simulink model "PID_spring_2mass_damper_system"  (R2022b)
settings: Solver=FixedStepAuto  StartTime=0  StopTime=Tf  FixedStep=dt  RelTol=1e-3
values from neighbouring files (symbols this model uses):
  c1 = 1    [P_2mass__slx_main.m]
  c2 = 2    [P_2mass__slx_main.m]
  control_on = true    [P_2mass__slx_main.m]
  f1 = 60    [P_2mass__slx_main.m]
  f2 = 30    [P_2mass__slx_main.m]
  k1 = 10    [P_2mass__slx_main.m]
  k2 = 20    [P_2mass__slx_main.m]
  m1 = 1    [P_2mass__slx_main.m]
  m2 = 5    [P_2mass__slx_main.m]
  r = [0 0 0 0]'    [P_2mass__slx_main.m]
  v1 = 0    [P_2mass__slx_main.m]
  v2 = 0    [P_2mass__slx_main.m]
  x1 = 1    [P_2mass__slx_main.m]
  x2 = 2    [P_2mass__slx_main.m]
settings Model: Creator=murayama  LastModifiedBy=murayama
settings DataIOCC: SaveFormat=StructureWithTime  ReturnWorkspaceOutputs=off
settings OptimizationCC: BlockReduction=off  BufferReuse=off
settings DebuggingCC: AlgebraicLoopMsg=none

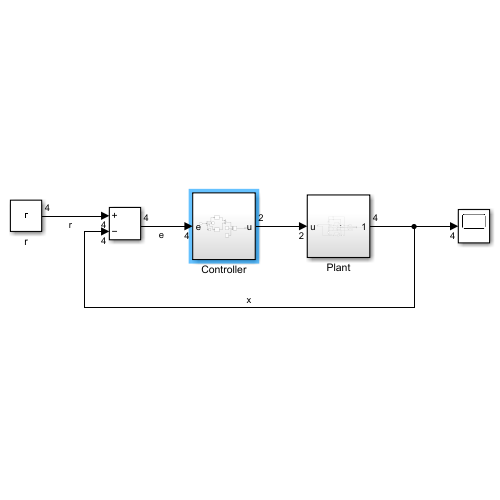
[thumbnail: Simulink's stored preview of the top-level diagram]
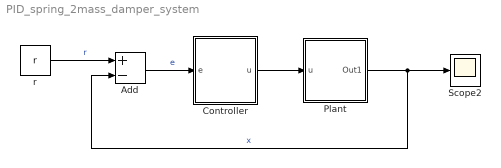
== system PID_spring_2mass_damper_system ==
  Add : Sum  Inputs=+-
  Controller : Subsystem
  Plant : Subsystem
  Scope2 : Scope
  r : Constant  Value=r
  wires:
  Plant/1(Out1) -> Scope2/1, Add/2  "x"
  r/1 -> Add/1  "r"
  Add/1 -> Controller/1(e)  "e"
  Controller/1(u) -> Plant/1(u)

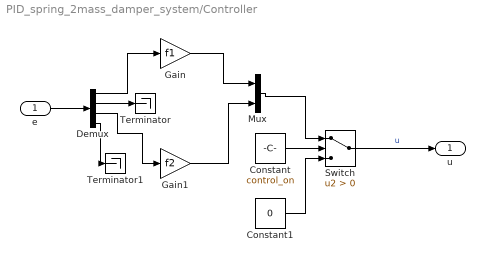
== system PID_spring_2mass_damper_system/Controller ==
  e : Inport
  Constant : Constant  Value=control_on
  Constant1 : Constant  Value=0
  Demux : Demux
  Gain : Gain  Gain=f1
  Gain1 : Gain  Gain=f2
  Mux : Mux  Inputs=2
  Switch : Switch  Criteria=u2 > Threshold  SaturateOnIntegerOverflow=off  InputSameDT=off
  Terminator : Terminator
  Terminator1 : Terminator
  u : Outport
  wires:
  Mux/1 -> Switch/1
  e/1 -> Demux/1
  Constant/1 -> Switch/2
  Switch/1 -> u/1  "u"
  Constant1/1 -> Switch/3
  Demux/1 -> Gain/1
  Gain/1 -> Mux/1
  Gain1/1 -> Mux/2
  Demux/2 -> Terminator/1
  Demux/4 -> Terminator1/1
  Demux/3 -> Gain1/1

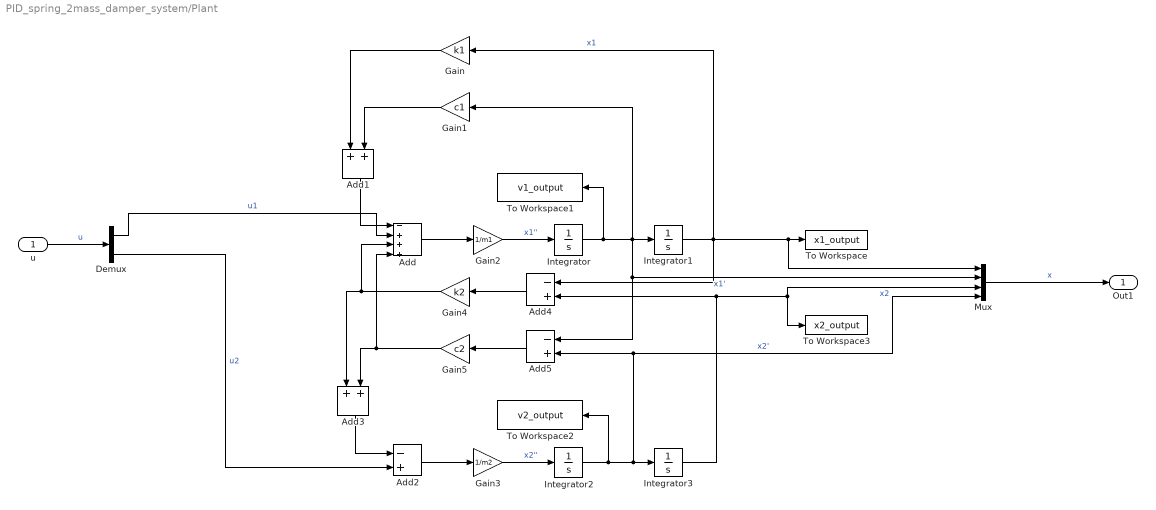
== system PID_spring_2mass_damper_system/Plant ==
  u : Inport
  Add : Sum  Inputs=-+++
  Add1 : Sum
  Add2 : Sum  Inputs=-+
  Add3 : Sum
  Add4 : Sum  Inputs=-+
  Add5 : Sum  Inputs=-+
  Demux : Demux  Outputs=2
  Gain : Gain  Gain=k1
  Gain1 : Gain  Gain=c1
  Gain2 : Gain  Gain=1/m1
  Gain3 : Gain  Gain=1/m2
  Gain4 : Gain  Gain=k2
  Gain5 : Gain  Gain=c2
  Integrator : Integrator  InitialCondition=v1
  Integrator1 : Integrator  InitialCondition=x1
  Integrator2 : Integrator  InitialCondition=v2
  Integrator3 : Integrator  InitialCondition=x2
  Mux : Mux
  To Workspace : ToWorkspace  VariableName=x1_output  SaveFormat=Timeseries  SampleTime=-1
  To Workspace1 : ToWorkspace  VariableName=v1_output  SaveFormat=Timeseries  SampleTime=-1
  To Workspace2 : ToWorkspace  VariableName=v2_output  SaveFormat=Timeseries  SampleTime=-1
  To Workspace3 : ToWorkspace  VariableName=x2_output  SaveFormat=Timeseries  SampleTime=-1
  Out1 : Outport
  wires:
  Integrator1/1 -> To Workspace/1, Mux/1, Gain/1, Add4/1  "x1"
  Add1/1 -> Add/1
  Gain/1 -> Add1/1
  Add/1 -> Gain2/1
  Gain2/1 -> Integrator/1  "x1''"
  Integrator/1 -> Add5/1, Mux/2, Gain1/1, Integrator1/1, To Workspace1/1  "x1'"
  Gain1/1 -> Add1/2
  Add2/1 -> Gain3/1
  Gain3/1 -> Integrator2/1  "x2''"
  Integrator2/1 -> To Workspace2/1, Mux/4, Add5/2, Integrator3/1  "x2'"
  Integrator3/1 -> Mux/3, To Workspace3/1, Add4/2  "x2"
  Gain4/1 -> Add3/1, Add/3
  Gain5/1 -> Add/4, Add3/2
  Add3/1 -> Add2/1
  Add4/1 -> Gain4/1
  Add5/1 -> Gain5/1
  Mux/1 -> Out1/1  "x"
  Demux/2 -> Add2/2  "u2"
  Demux/1 -> Add/2  "u1"
  u/1 -> Demux/1  "u"
